simulink model "Drag_Model_V"  (R2020b)
settings: Solver=VariableStepAuto  StartTime=0.0  StopTime=10.0  RelTol=1e-3
values from neighbouring files (symbols this model uses):
  C_D = 0.6    [ANGULARTUNEVERSION2_VandV.m]    (also in Drag_Model_VV.m)
  rho = 1.225    [ANGULARTUNEVERSION2_VandV.m]    (also in Drag_Model_VV.m)
  S = 1*1.8    (= 1.8)    [ANGULARTUNEVERSION2_VandV.m]    (also in Drag_Model_VV.m = 2.5)
  v_gust = [1; 2; 3]    [Drag_Model_VV.m]
  v_vehicle = [20; 10; 0]    [ANGULARTUNEVERSION2_VandV.m]    (also in Drag_Model_VV.m = [2;3;4])
settings Model: Creator=Jonathan van Zyl  LastModifiedBy=Jonathan van Zyl

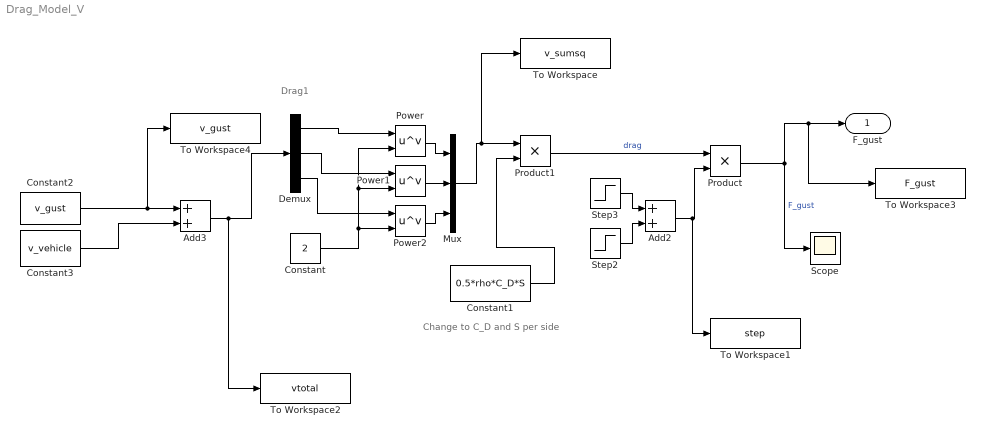
== system Drag_Model_V ==
  note: Change to C_D and S per side
  note: Drag1
  Add2 : Sum
  Add3 : Sum
  Constant : Constant  Value=2
  Constant1 : Constant  Value=0.5*rho*C_D*S
  Constant2 : Constant  Value=v_gust
  Constant3 : Constant  Value=v_vehicle
  Demux : Demux  Outputs=3
  Mux : Mux  Inputs=3
  Power : Math  Operator=pow  SaturateOnIntegerOverflow=on
  Power1 : Math  Operator=pow  SaturateOnIntegerOverflow=on
  Power2 : Math  Operator=pow  SaturateOnIntegerOverflow=on
  Product : Product
  Product1 : Product
  Scope : Scope
  Step2 : Step  Time=0  SampleTime=0
  Step3 : Step  Time=10.5  After=-1  SampleTime=0
  To Workspace : ToWorkspace  VariableName=v_sumsq  SampleTime=-1
  To Workspace1 : ToWorkspace  VariableName=step  SaveFormat=Timeseries  SampleTime=-1
  To Workspace2 : ToWorkspace  VariableName=vtotal  SaveFormat=Timeseries  SampleTime=-1
  To Workspace3 : ToWorkspace  VariableName=F_gust  SaveFormat=Timeseries  SampleTime=-1
  To Workspace4 : ToWorkspace  VariableName=v_gust  SaveFormat=Timeseries  SampleTime=-1
  F_gust : Outport
  wires:
  Step3/1 -> Add2/1
  Product/1 -> To Workspace3/1, F_gust/1, Scope/1  "F_gust"
  Constant2/1 -> To Workspace4/1, Add3/1
  Add2/1 -> To Workspace1/1, Product/2
  Mux/1 -> To Workspace/1, Product1/1
  Power2/1 -> Mux/3
  Add3/1 -> To Workspace2/1, Demux/1
  Product1/1 -> Product/1  "drag"
  Constant1/1 -> Product1/2
  Demux/3 -> Power2/1
  Step2/1 -> Add2/2
  Power1/1 -> Mux/2
  Power/1 -> Mux/1
  Demux/2 -> Power1/1
  Constant3/1 -> Add3/2
  Constant/1 -> Power2/2, Power1/2, Power/2
  Demux/1 -> Power/1
